simulink library "ammclib_bam_S32K14x"  (R2016a)
settings: Solver=VariableStepAuto  SolverMode=SingleTasking  StartTime=0.0  StopTime=10.0  RelTol=1e-3
undefined symbols (not defined in the file or in its folder): f16A1, f16A2, f16ADCMaxError, f16B0, f16B1, f16B2, f16C1, f16CC1, f16CC1sc, f16CC1sc_D, f16CC1sc_Q, f16CC2, f16CC2sc, f16CC2sc_D, f16CC2sc_Q, f16DerivGain, f16EGain, f16FiltCoef, f16HystOff, f16HystOn, f16IGain, f16IntegGain, f16IntegGainFW, f16IntegGainQ, f16Kd, f16Kq, f16Limit, f16LowerLimit, f16LowerLimit_D, f16LowerLimit_Q, f16LowerLimitFW, f16LowerLimitQ, f16ModIndex, f16OutValOff, f16OutValOn, f16PropGain, f16PropGainFW, f16PropGainQ, f16RampDown, f16RampUp, f16UGain, f16UpperLimit, f16UpperLimit_D, f16UpperLimit_Q, f16UpperLimitFW, f16UpperLimitQ, f16WIGain, f32A1, f32A2, f32ADCMaxError, f32B0, f32B1, f32B2, f32C1, f32CC1, f32CC1sc, f32CC1sc_D, f32CC1sc_Q, f32CC2, f32CC2sc ... (+114)
(part 16 of 22)

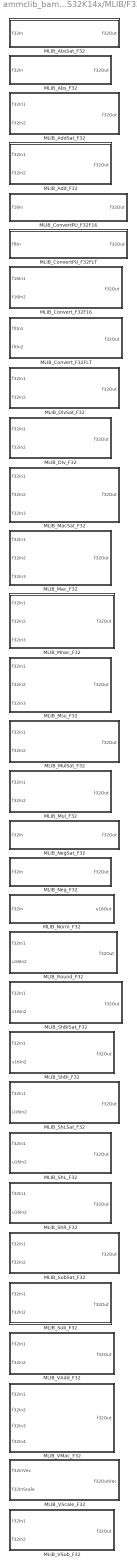
== system ammclib_bam_S32K14x/MLIB/F32 ==
  MLIB_AbsSat_F32 : Subsystem  TreatAsAtomicUnit=on  mask(MLIB_AbsSat_F32){}
      mask help: Saturated absolute value in 32-bit fixed-point fractional implementation. Refer to the AMMCLIB User's Guide for further details.
      mask init: same as ammclib_bam_S32K14x/GDFLIB/F16/GDFLIB_FilterFIR_F16
      settings: RTWSystemCode=Inline
      mask Help: web([fileparts(which('ammclib_bam_S32K14x.slx')) '/../doc/S32K14XMCLUG.pdf'], '-browser')
      mask Display: pos = get_param(gcb, 'Position');width = pos(3) - pos(1); height = pos(4) - pos(2);tX=width/2;tY=height - 8;color('black');text(tX,tY, 'MLIB_AbsSat_F32', 'horizontalAlignment', 'center');
  MLIB_Abs_F32 : Subsystem  TreatAsAtomicUnit=on  mask(MLIB_Abs_F32){}
      mask help: Unsaturated absolute value in 32-bit fixed-point fractional implementation. Refer to the AMMCLIB User's Guide for further details.
      mask init: same as ammclib_bam_S32K14x/GDFLIB/F16/GDFLIB_FilterFIR_F16
      settings: RTWSystemCode=Inline
      mask Help: web([fileparts(which('ammclib_bam_S32K14x.slx')) '/../doc/S32K14XMCLUG.pdf'], '-browser')
      mask Display: pos = get_param(gcb, 'Position');width = pos(3) - pos(1); height = pos(4) - pos(2);tX=width/2;tY=height - 8;color('black');text(tX,tY, 'MLIB_Abs_F32', 'horizontalAlignment', 'center');
  MLIB_AddSat_F32 : Subsystem  TreatAsAtomicUnit=on  mask(MLIB_AddSat_F32){}
      mask help: Saturated addition in 32-bit fixed-point fractional implementation. Refer to the AMMCLIB User's Guide for further details.
      mask init: same as ammclib_bam_S32K14x/GDFLIB/F16/GDFLIB_FilterFIR_F16
      settings: RTWSystemCode=Inline
      mask Help: web([fileparts(which('ammclib_bam_S32K14x.slx')) '/../doc/S32K14XMCLUG.pdf'], '-browser')
      mask Display: pos = get_param(gcb, 'Position');width = pos(3) - pos(1); height = pos(4) - pos(2);tX=width/2;tY=height - 8;color('black');text(tX,tY, 'MLIB_AddSat_F32', 'horizontalAlignment', 'center');
  MLIB_Add_F32 : Subsystem  TreatAsAtomicUnit=on  mask(MLIB_Add_F32){}
      mask help: Unsaturated addition in 32-bit fixed-point fractional implementation.
      mask init: same as ammclib_bam_S32K14x/GDFLIB/F16/GDFLIB_FilterFIR_F16
      settings: RTWSystemCode=Inline
      mask Help: web([fileparts(which('ammclib_bam_S32K14x.slx')) '/../doc/S32K14XMCLUG.pdf'], '-browser')
      mask Display: pos = get_param(gcb, 'Position');width = pos(3) - pos(1); height = pos(4) - pos(2);tX=width/2;tY=height - 8;color('black');text(tX,tY, 'MLIB_Add_F32', 'horizontalAlignment', 'center');
  MLIB_ConvertPU_F32F16 : Subsystem  TreatAsAtomicUnit=on  mask(MLIB_ConvertPU_F32F16){}
      mask help: Conversion of a 16-bit fixed-point fractional value to a 32-bit fixed-point fractional equivalent. Refer to the AMMCLIB User's Guide for further details.
      mask init: same as ammclib_bam_S32K14x/GDFLIB/F16/GDFLIB_FilterFIR_F16
      settings: RTWSystemCode=Inline
      mask Help: web([fileparts(which('ammclib_bam_S32K14x.slx')) '/../doc/S32K14XMCLUG.pdf'], '-browser')
      mask Display: pos = get_param(gcb, 'Position');width = pos(3) - pos(1); height = pos(4) - pos(2);tX=width/2;tY=height - 8;color('black');text(tX,tY, 'MLIB_ConvertPU_F32F16', 'horizontalAlignment', 'center');
  MLIB_ConvertPU_F32FLT : Subsystem  TreatAsAtomicUnit=on  mask(MLIB_ConvertPU_F32FLT){}
      mask help: Conversion of a single precision floating-point value to a 32-bit fixed-point fractional equivalent. Refer to the AMMCLIB User's Guide for further details.
      mask init: same as ammclib_bam_S32K14x/GDFLIB/F16/GDFLIB_FilterFIR_F16
      settings: RTWSystemCode=Inline
      mask Help: web([fileparts(which('ammclib_bam_S32K14x.slx')) '/../doc/S32K14XMCLUG.pdf'], '-browser')
      mask Display: pos = get_param(gcb, 'Position');width = pos(3) - pos(1); height = pos(4) - pos(2);tX=width/2;tY=height - 8;color('black');text(tX,tY, 'MLIB_ConvertPU_F32FLT', 'horizontalAlignment', 'center');
  MLIB_Convert_F32F16 : Subsystem  TreatAsAtomicUnit=on  mask(MLIB_Convert_F32F16){}
      mask help: Scaled conversion of a 16-bit fixed-point fractional value to a 32-bit fixed-point fractional equivalent. Refer to the AMMCLIB User's Guide for further details.
      mask init: same as ammclib_bam_S32K14x/GDFLIB/F16/GDFLIB_FilterFIR_F16
      settings: RTWSystemCode=Inline
      mask Help: web([fileparts(which('ammclib_bam_S32K14x.slx')) '/../doc/S32K14XMCLUG.pdf'], '-browser')
      mask Display: pos = get_param(gcb, 'Position');width = pos(3) - pos(1); height = pos(4) - pos(2);tX=width/2;tY=height - 8;color('black');text(tX,tY, 'MLIB_Convert_F32F16', 'horizontalAlignment', 'center');
  MLIB_Convert_F32FLT : Subsystem  TreatAsAtomicUnit=on  mask(MLIB_Convert_F32FLT){}
      mask help: Scaled conversion of a single precision floating-point value to a 32-bit fixed-point fractional equivalent. Refer to the AMMCLIB User's Guide for further details.
      mask init: same as ammclib_bam_S32K14x/GDFLIB/F16/GDFLIB_FilterFIR_F16
      settings: RTWSystemCode=Inline
      mask Help: web([fileparts(which('ammclib_bam_S32K14x.slx')) '/../doc/S32K14XMCLUG.pdf'], '-browser')
      mask Display: pos = get_param(gcb, 'Position');width = pos(3) - pos(1); height = pos(4) - pos(2);tX=width/2;tY=height - 8;color('black');text(tX,tY, 'MLIB_Convert_F32FLT', 'horizontalAlignment', 'center');
  MLIB_DivSat_F32 : Subsystem  TreatAsAtomicUnit=on  mask(MLIB_DivSat_F32){}
      mask help: Saturated division of two input values in 32-bit fixed-point fractional implementation. Refer to the AMMCLIB User's Guide for further details.
      mask init: same as ammclib_bam_S32K14x/GDFLIB/F16/GDFLIB_FilterFIR_F16
      settings: RTWSystemCode=Inline
      mask Help: web([fileparts(which('ammclib_bam_S32K14x.slx')) '/../doc/S32K14XMCLUG.pdf'], '-browser')
      mask Display: pos = get_param(gcb, 'Position');width = pos(3) - pos(1); height = pos(4) - pos(2);tX=width/2;tY=height - 8;color('black');text(tX,tY, 'MLIB_DivSat_F32', 'horizontalAlignment', 'center');
  MLIB_Div_F32 : Subsystem  TreatAsAtomicUnit=on  mask(MLIB_Div_F32){}
      mask help: Division of two input values without saturation in 32-bit fixed-point fractional implementation. Refer to the AMMCLIB User's Guide for further details.
      mask init: same as ammclib_bam_S32K14x/GDFLIB/F16/GDFLIB_FilterFIR_F16
      settings: RTWSystemCode=Inline
      mask Help: web([fileparts(which('ammclib_bam_S32K14x.slx')) '/../doc/S32K14XMCLUG.pdf'], '-browser')
      mask Display: pos = get_param(gcb, 'Position');width = pos(3) - pos(1); height = pos(4) - pos(2);tX=width/2;tY=height - 8;color('black');text(tX,tY, 'MLIB_Div_F32', 'horizontalAlignment', 'center');
  MLIB_MacSat_F32 : Subsystem  TreatAsAtomicUnit=on  mask(MLIB_MacSat_F32){}
      mask help: Saturated multiply-accumulate of input values in 32-bit fixed-point fractional implementation. Refer to the AMMCLIB User's Guide for further details.
      mask init: same as ammclib_bam_S32K14x/GDFLIB/F16/GDFLIB_FilterFIR_F16
      settings: RTWSystemCode=Inline
      mask Help: web([fileparts(which('ammclib_bam_S32K14x.slx')) '/../doc/S32K14XMCLUG.pdf'], '-browser')
      mask Display: pos = get_param(gcb, 'Position');width = pos(3) - pos(1); height = pos(4) - pos(2);tX=width/2;tY=height - 8;color('black');text(tX,tY, 'MLIB_MacSat_F32', 'horizontalAlignment', 'center');
  MLIB_Mac_F32 : Subsystem  TreatAsAtomicUnit=on  mask(MLIB_Mac_F32){}
      mask help: Unsaturated multiply-accumulate function in 32-bit fixed-point fractional implementation. Refer to the AMMCLIB User's Guide for further details.
      mask init: same as ammclib_bam_S32K14x/GDFLIB/F16/GDFLIB_FilterFIR_F16
      settings: RTWSystemCode=Inline
      mask Help: web([fileparts(which('ammclib_bam_S32K14x.slx')) '/../doc/S32K14XMCLUG.pdf'], '-browser')
      mask Display: pos = get_param(gcb, 'Position');width = pos(3) - pos(1); height = pos(4) - pos(2);tX=width/2;tY=height - 8;color('black');text(tX,tY, 'MLIB_Mac_F32', 'horizontalAlignment', 'center');
  MLIB_Mnac_F32 : Subsystem  TreatAsAtomicUnit=on  mask(MLIB_Mnac_F32){}
      mask help: Unsaturated multiply-negative-accumulate function in 32-bit fixed-point fractional implementation. Refer to the AMMCLIB User's Guide for further details.
      mask init: same as ammclib_bam_S32K14x/GDFLIB/F16/GDFLIB_FilterFIR_F16
      settings: RTWSystemCode=Inline
      mask Help: web([fileparts(which('ammclib_bam_S32K14x.slx')) '/../doc/S32K14XMCLUG.pdf'], '-browser')
      mask Display: pos = get_param(gcb, 'Position');width = pos(3) - pos(1); height = pos(4) - pos(2);tX=width/2;tY=height - 8;color('black');text(tX,tY, 'MLIB_Mnac_F32', 'horizontalAlignment', 'center');
  MLIB_Msu_F32 : Subsystem  TreatAsAtomicUnit=on  mask(MLIB_Msu_F32){}
      mask help: Unsaturated multiply-subtract-from function in 32-bit fixed-point fractional implementation. Refer to the AMMCLIB User's Guide for further details.
      mask init: same as ammclib_bam_S32K14x/GDFLIB/F16/GDFLIB_FilterFIR_F16
      settings: RTWSystemCode=Inline
      mask Help: web([fileparts(which('ammclib_bam_S32K14x.slx')) '/../doc/S32K14XMCLUG.pdf'], '-browser')
      mask Display: pos = get_param(gcb, 'Position');width = pos(3) - pos(1); height = pos(4) - pos(2);tX=width/2;tY=height - 8;color('black');text(tX,tY, 'MLIB_Msu_F32', 'horizontalAlignment', 'center');
  MLIB_MulSat_F32 : Subsystem  TreatAsAtomicUnit=on  mask(MLIB_MulSat_F32){}
      mask help: Saturated multiplication of two input values in 32-bit fixed-point fractional implementation. Refer to the AMMCLIB User's Guide for further details.
      mask init: same as ammclib_bam_S32K14x/GDFLIB/F16/GDFLIB_FilterFIR_F16
      settings: RTWSystemCode=Inline
      mask Help: web([fileparts(which('ammclib_bam_S32K14x.slx')) '/../doc/S32K14XMCLUG.pdf'], '-browser')
      mask Display: pos = get_param(gcb, 'Position');width = pos(3) - pos(1); height = pos(4) - pos(2);tX=width/2;tY=height - 8;color('black');text(tX,tY, 'MLIB_MulSat_F32', 'horizontalAlignment', 'center');
  MLIB_Mul_F32 : Subsystem  TreatAsAtomicUnit=on  mask(MLIB_Mul_F32){}
      mask help: Unsaturated multiplication of two input values in 32-bit fixed-point fractional implementation. Refer to the AMMCLIB User's Guide for further details.
      mask init: same as ammclib_bam_S32K14x/GDFLIB/F16/GDFLIB_FilterFIR_F16
      settings: RTWSystemCode=Inline
      mask Help: web([fileparts(which('ammclib_bam_S32K14x.slx')) '/../doc/S32K14XMCLUG.pdf'], '-browser')
      mask Display: pos = get_param(gcb, 'Position');width = pos(3) - pos(1); height = pos(4) - pos(2);tX=width/2;tY=height - 8;color('black');text(tX,tY, 'MLIB_Mul_F32', 'horizontalAlignment', 'center');
  MLIB_NegSat_F32 : Subsystem  TreatAsAtomicUnit=on  mask(MLIB_NegSat_F32){}
      mask help: Saturated negation in 32-bit fixed-point fractional implementation. Refer to the AMMCLIB User's Guide for further details.
      mask init: same as ammclib_bam_S32K14x/GDFLIB/F16/GDFLIB_FilterFIR_F16
      settings: RTWSystemCode=Inline
      mask Help: web([fileparts(which('ammclib_bam_S32K14x.slx')) '/../doc/S32K14XMCLUG.pdf'], '-browser')
      mask Display: pos = get_param(gcb, 'Position');width = pos(3) - pos(1); height = pos(4) - pos(2);tX=width/2;tY=height - 8;color('black');text(tX,tY, 'MLIB_NegSat_F32', 'horizontalAlignment', 'center');
  MLIB_Neg_F32 : Subsystem  TreatAsAtomicUnit=on  mask(MLIB_Neg_F32){}
      mask help: Unsaturated negation in 32-bit fixed-point fractional implementation. Refer to the AMMCLIB User's Guide for further details.
      mask init: same as ammclib_bam_S32K14x/GDFLIB/F16/GDFLIB_FilterFIR_F16
      settings: RTWSystemCode=Inline
      mask Help: web([fileparts(which('ammclib_bam_S32K14x.slx')) '/../doc/S32K14XMCLUG.pdf'], '-browser')
      mask Display: pos = get_param(gcb, 'Position');width = pos(3) - pos(1); height = pos(4) - pos(2);tX=width/2;tY=height - 8;color('black');text(tX,tY, 'MLIB_Neg_F32', 'horizontalAlignment', 'center');
  MLIB_Norm_F32 : Subsystem  TreatAsAtomicUnit=on  mask(MLIB_Norm_F32){}
      mask help: Normalization function in 32-bit fixed-point fractional implementation. The function counts the number of left shift needed for normalization of the input fractional value. Refer to the AMMCLIB User's Guide for further details.
      mask init: same as ammclib_bam_S32K14x/GDFLIB/F16/GDFLIB_FilterFIR_F16
      settings: RTWSystemCode=Inline
      mask Help: web([fileparts(which('ammclib_bam_S32K14x.slx')) '/../doc/S32K14XMCLUG.pdf'], '-browser')
      mask Display: pos = get_param(gcb, 'Position');width = pos(3) - pos(1); height = pos(4) - pos(2);tX=width/2;tY=height - 8;color('black');text(tX,tY, 'MLIB_Norm_F32', 'horizontalAlignment', 'center');
  MLIB_Round_F32 : Subsystem  TreatAsAtomicUnit=on  mask(MLIB_Round_F32){}
      mask help: Rounding function in 32-bit fixed-point fractional implementation. The function rounds the first input value to the number of digits defined by second input value and saturates the result. Refer to the AMMCLIB User's Guide for further details.
      mask init: same as ammclib_bam_S32K14x/GDFLIB/F16/GDFLIB_FilterFIR_F16
      settings: RTWSystemCode=Inline
      mask Help: web([fileparts(which('ammclib_bam_S32K14x.slx')) '/../doc/S32K14XMCLUG.pdf'], '-browser')
      mask Display: pos = get_param(gcb, 'Position');width = pos(3) - pos(1); height = pos(4) - pos(2);tX=width/2;tY=height - 8;color('black');text(tX,tY, 'MLIB_Round_F32', 'horizontalAlignment', 'center');
  MLIB_ShBiSat_F32 : Subsystem  TreatAsAtomicUnit=on  mask(MLIB_ShBiSat_F32){}
      mask help: Saturated bidirectional shift in 32-bit fixed-point fractional implementation. The function shifts the first input value to the left (if the second input is negative) or right (if the second input is positive) by the amount defined by second input value, saturating the result. Refer to the AMMCLIB User's Guide for further details.
      mask init: same as ammclib_bam_S32K14x/GDFLIB/F16/GDFLIB_FilterFIR_F16
      settings: RTWSystemCode=Inline
      mask Help: web([fileparts(which('ammclib_bam_S32K14x.slx')) '/../doc/S32K14XMCLUG.pdf'], '-browser')
      mask Display: pos = get_param(gcb, 'Position');width = pos(3) - pos(1); height = pos(4) - pos(2);tX=width/2;tY=height - 8;color('black');text(tX,tY, 'MLIB_ShBiSat_F32', 'horizontalAlignment', 'center');
  MLIB_ShBi_F32 : Subsystem  TreatAsAtomicUnit=on  mask(MLIB_ShBi_F32){}
      mask help: Unsaturated bidirectional shift in 32-bit fixed-point fractional implementation. The function shifts the first input value to the left (if the second input is negative) or right (if the second input is positive) by the amount defined by second input value. Refer to the AMMCLIB User's Guide for further details.
      mask init: same as ammclib_bam_S32K14x/GDFLIB/F16/GDFLIB_FilterFIR_F16
      settings: RTWSystemCode=Inline
      mask Help: web([fileparts(which('ammclib_bam_S32K14x.slx')) '/../doc/S32K14XMCLUG.pdf'], '-browser')
      mask Display: pos = get_param(gcb, 'Position');width = pos(3) - pos(1); height = pos(4) - pos(2);tX=width/2;tY=height - 8;color('black');text(tX,tY, 'MLIB_ShBi_F32', 'horizontalAlignment', 'center');
  MLIB_ShLSat_F32 : Subsystem  TreatAsAtomicUnit=on  mask(MLIB_ShLSat_F32){}
      mask help: Saturated shift left in 32-bit fixed-point fractional implementation. The function shifts the first input value to the left by the amount defined by the second input value, saturating the result. Refer to the AMMCLIB User's Guide for further details.
      mask init: same as ammclib_bam_S32K14x/GDFLIB/F16/GDFLIB_FilterFIR_F16
      settings: RTWSystemCode=Inline
      mask Help: web([fileparts(which('ammclib_bam_S32K14x.slx')) '/../doc/S32K14XMCLUG.pdf'], '-browser')
      mask Display: pos = get_param(gcb, 'Position');width = pos(3) - pos(1); height = pos(4) - pos(2);tX=width/2;tY=height - 8;color('black');text(tX,tY, 'MLIB_ShLSat_F32', 'horizontalAlignment', 'center');
  MLIB_ShL_F32 : Subsystem  TreatAsAtomicUnit=on  mask(MLIB_ShL_F32){}
      mask help: Unsaturated shift left in 32-bit fixed-point fractional implementation. The function shifts the first input value to the left by the amount defined by the second input value. Refer to the AMMCLIB User's Guide for further details.
      mask init: same as ammclib_bam_S32K14x/GDFLIB/F16/GDFLIB_FilterFIR_F16
      settings: RTWSystemCode=Inline
      mask Help: web([fileparts(which('ammclib_bam_S32K14x.slx')) '/../doc/S32K14XMCLUG.pdf'], '-browser')
      mask Display: pos = get_param(gcb, 'Position');width = pos(3) - pos(1); height = pos(4) - pos(2);tX=width/2;tY=height - 8;color('black');text(tX,tY, 'MLIB_ShL_F32', 'horizontalAlignment', 'center');
  MLIB_ShR_F32 : Subsystem  TreatAsAtomicUnit=on  mask(MLIB_ShR_F32){}
      mask help: Unsaturated shift right in 32-bit fixed-point fractional implementation. The function shifts the first input value to the right by the amount defined by the second input value. Refer to the AMMCLIB User's Guide for further details.
      mask init: same as ammclib_bam_S32K14x/GDFLIB/F16/GDFLIB_FilterFIR_F16
      settings: RTWSystemCode=Inline
      mask Help: web([fileparts(which('ammclib_bam_S32K14x.slx')) '/../doc/S32K14XMCLUG.pdf'], '-browser')
      mask Display: pos = get_param(gcb, 'Position');width = pos(3) - pos(1); height = pos(4) - pos(2);tX=width/2;tY=height - 8;color('black');text(tX,tY, 'MLIB_ShR_F32', 'horizontalAlignment', 'center');
  MLIB_SubSat_F32 : Subsystem  TreatAsAtomicUnit=on  mask(MLIB_SubSat_F32){}
      mask help: Saturated subtraction in 32-bit fixed-point fractional implementation. Refer to the AMMCLIB User's Guide for further details.
      mask init: same as ammclib_bam_S32K14x/GDFLIB/F16/GDFLIB_FilterFIR_F16
      settings: RTWSystemCode=Inline
      mask Help: web([fileparts(which('ammclib_bam_S32K14x.slx')) '/../doc/S32K14XMCLUG.pdf'], '-browser')
      mask Display: pos = get_param(gcb, 'Position');width = pos(3) - pos(1); height = pos(4) - pos(2);tX=width/2;tY=height - 8;color('black');text(tX,tY, 'MLIB_SubSat_F32', 'horizontalAlignment', 'center');
  MLIB_Sub_F32 : Subsystem  TreatAsAtomicUnit=on  mask(MLIB_Sub_F32){}
      mask help: Unsaturated subtraction in 32-bit fixed-point fractional implementation. Refer to the AMMCLIB User's Guide for further details.
      mask init: same as ammclib_bam_S32K14x/GDFLIB/F16/GDFLIB_FilterFIR_F16
      settings: RTWSystemCode=Inline
      mask Help: web([fileparts(which('ammclib_bam_S32K14x.slx')) '/../doc/S32K14XMCLUG.pdf'], '-browser')
      mask Display: pos = get_param(gcb, 'Position');width = pos(3) - pos(1); height = pos(4) - pos(2);tX=width/2;tY=height - 8;color('black');text(tX,tY, 'MLIB_Sub_F32', 'horizontalAlignment', 'center');
  MLIB_VAdd_F32 : Subsystem  TreatAsAtomicUnit=on  mask(MLIB_VAdd_F32){}
      mask help: Vector addition in 32-bit fixed-point fractional implementation.
      mask init: same as ammclib_bam_S32K14x/GDFLIB/F16/GDFLIB_FilterFIR_F16
      settings: RTWSystemCode=Inline
      mask Help: web([fileparts(which('ammclib_bam_S32K14x.slx')) '/../doc/S32K14XMCLUG.pdf'], '-browser')
      mask Display: pos = get_param(gcb, 'Position');width = pos(3) - pos(1); height = pos(4) - pos(2);tX=width/2;tY=height - 8;color('black');text(tX,tY, 'MLIB_VAdd_F32', 'horizontalAlignment', 'center');
  MLIB_VMac_F32 : Subsystem  TreatAsAtomicUnit=on  mask(MLIB_VMac_F32){}
      mask help: Dot product of 2-element vectors with saturated multiplication and modulo accumulation in 32-bit fixed-point fractional implementation. Refer to the AMMCLIB User's Guide for further details.
      mask init: same as ammclib_bam_S32K14x/GDFLIB/F16/GDFLIB_FilterFIR_F16
      settings: RTWSystemCode=Inline
      mask Help: web([fileparts(which('ammclib_bam_S32K14x.slx')) '/../doc/S32K14XMCLUG.pdf'], '-browser')
      mask Display: pos = get_param(gcb, 'Position');width = pos(3) - pos(1); height = pos(4) - pos(2);tX=width/2;tY=height - 8;color('black');text(tX,tY, 'MLIB_VMac_F32', 'horizontalAlignment', 'center');
  MLIB_VScale_F32 : Subsystem  TreatAsAtomicUnit=on  mask(MLIB_VScale_F32){}
      mask help: Multiplication of a vector and scalar in 32-bit fixed-point fractional implementation.
      mask init: same as ammclib_bam_S32K14x/GDFLIB/F16/GDFLIB_FilterFIR_F16
      settings: RTWSystemCode=Inline
      mask Help: web([fileparts(which('ammclib_bam_S32K14x.slx')) '/../doc/S32K14XMCLUG.pdf'], '-browser')
      mask Display: pos = get_param(gcb, 'Position');width = pos(3) - pos(1); height = pos(4) - pos(2);tX=width/2;tY=height - 8;color('black');text(tX,tY, 'MLIB_VScale_F32', 'horizontalAlignment', 'center');
  MLIB_VSub_F32 : Subsystem  TreatAsAtomicUnit=on  mask(MLIB_VSub_F32){}
      mask help: Vector substraction in 32-bit fixed-point fractional implementation.
      mask init: same as ammclib_bam_S32K14x/GDFLIB/F16/GDFLIB_FilterFIR_F16
      settings: RTWSystemCode=Inline
      mask Help: web([fileparts(which('ammclib_bam_S32K14x.slx')) '/../doc/S32K14XMCLUG.pdf'], '-browser')
      mask Display: pos = get_param(gcb, 'Position');width = pos(3) - pos(1); height = pos(4) - pos(2);tX=width/2;tY=height - 8;color('black');text(tX,tY, 'MLIB_VSub_F32', 'horizontalAlignment', 'center');

== system ammclib_bam_S32K14x/MLIB/F32F16F16 ==
  MLIB_MacSat_F32F16F16 : Subsystem  TreatAsAtomicUnit=on  mask(MLIB_MacSat_F32F16F16){}
      mask help: Saturated multiply-accumulate of input values in 16/32-bit fixed-point fractional implementation. Refer to the AMMCLIB User's Guide for further details.
      mask init: same as ammclib_bam_S32K14x/GDFLIB/F16/GDFLIB_FilterFIR_F16
      settings: RTWSystemCode=Inline
      mask Help: web([fileparts(which('ammclib_bam_S32K14x.slx')) '/../doc/S32K14XMCLUG.pdf'], '-browser')
      mask Display: pos = get_param(gcb, 'Position');width = pos(3) - pos(1); height = pos(4) - pos(2);tX=width/2;tY=height - 8;color('black');text(tX,tY, 'MLIB_MacSat_F32F16F16', 'horizontalAlignment', 'center');
  MLIB_Mac_F32F16F16 : Subsystem  TreatAsAtomicUnit=on  mask(MLIB_Mac_F32F16F16){}
      mask help: Unsaturated multiply-accumulate function in 16/32-bit fixed-point fractional implementation. Refer to the AMMCLIB User's Guide for further details.
      mask init: same as ammclib_bam_S32K14x/GDFLIB/F16/GDFLIB_FilterFIR_F16
      settings: RTWSystemCode=Inline
      mask Help: web([fileparts(which('ammclib_bam_S32K14x.slx')) '/../doc/S32K14XMCLUG.pdf'], '-browser')
      mask Display: pos = get_param(gcb, 'Position');width = pos(3) - pos(1); height = pos(4) - pos(2);tX=width/2;tY=height - 8;color('black');text(tX,tY, 'MLIB_Mac_F32F16F16', 'horizontalAlignment', 'center');
  MLIB_Mnac_F32F16F16 : Subsystem  TreatAsAtomicUnit=on  mask(MLIB_Mnac_F32F16F16){}
      mask help: Unsaturated multiply-negative-accumulate function in 16/32-bit fixed-point fractional implementation. Refer to the AMMCLIB User's Guide for further details.
      mask init: same as ammclib_bam_S32K14x/GDFLIB/F16/GDFLIB_FilterFIR_F16
      settings: RTWSystemCode=Inline
      mask Help: web([fileparts(which('ammclib_bam_S32K14x.slx')) '/../doc/S32K14XMCLUG.pdf'], '-browser')
      mask Display: pos = get_param(gcb, 'Position');width = pos(3) - pos(1); height = pos(4) - pos(2);tX=width/2;tY=height - 8;color('black');text(tX,tY, 'MLIB_Mnac_F32F16F16', 'horizontalAlignment', 'center');
  MLIB_Msu_F32F16F16 : Subsystem  TreatAsAtomicUnit=on  mask(MLIB_Msu_F32F16F16){}
      mask help: Unsaturated multiply-subtract-from function in 16/32-bit fixed-point fractional implementation. Refer to the AMMCLIB User's Guide for further details.
      mask init: same as ammclib_bam_S32K14x/GDFLIB/F16/GDFLIB_FilterFIR_F16
      settings: RTWSystemCode=Inline
      mask Help: web([fileparts(which('ammclib_bam_S32K14x.slx')) '/../doc/S32K14XMCLUG.pdf'], '-browser')
      mask Display: pos = get_param(gcb, 'Position');width = pos(3) - pos(1); height = pos(4) - pos(2);tX=width/2;tY=height - 8;color('black');text(tX,tY, 'MLIB_Msu_F32F16F16', 'horizontalAlignment', 'center');
  MLIB_MulSat_F32F16F16 : Subsystem  TreatAsAtomicUnit=on  mask(MLIB_MulSat_F32F16F16){}
      mask help: Saturated multiplication of two input values in 16/32-bit fixed-point fractional implementation. Refer to the AMMCLIB User's Guide for further details.
      mask init: same as ammclib_bam_S32K14x/GDFLIB/F16/GDFLIB_FilterFIR_F16
      settings: RTWSystemCode=Inline
      mask Help: web([fileparts(which('ammclib_bam_S32K14x.slx')) '/../doc/S32K14XMCLUG.pdf'], '-browser')
      mask Display: pos = get_param(gcb, 'Position');width = pos(3) - pos(1); height = pos(4) - pos(2);tX=width/2;tY=height - 8;color('black');text(tX,tY, 'MLIB_MulSat_F32F16F16', 'horizontalAlignment', 'center');
  MLIB_Mul_F32F16F16 : Subsystem  TreatAsAtomicUnit=on  mask(MLIB_Mul_F32F16F16){}
      mask help: Unsaturated multiplication of two input values in 16/32-bit fixed-point fractional implementation. Refer to the AMMCLIB User's Guide for further details.
      mask init: same as ammclib_bam_S32K14x/GDFLIB/F16/GDFLIB_FilterFIR_F16
      settings: RTWSystemCode=Inline
      mask Help: web([fileparts(which('ammclib_bam_S32K14x.slx')) '/../doc/S32K14XMCLUG.pdf'], '-browser')
      mask Display: pos = get_param(gcb, 'Position');width = pos(3) - pos(1); height = pos(4) - pos(2);tX=width/2;tY=height - 8;color('black');text(tX,tY, 'MLIB_Mul_F32F16F16', 'horizontalAlignment', 'center');
  MLIB_VMac_F32F16F16 : Subsystem  TreatAsAtomicUnit=on  mask(MLIB_VMac_F32F16F16){}
      mask help: Dot product of 2-element vectors with saturated multiplication and modulo accumulation in 16/32-bit fixed-point fractional implementation. Refer to the AMMCLIB User's Guide for further details.
      mask init: same as ammclib_bam_S32K14x/GDFLIB/F16/GDFLIB_FilterFIR_F16
      settings: RTWSystemCode=Inline
      mask Help: web([fileparts(which('ammclib_bam_S32K14x.slx')) '/../doc/S32K14XMCLUG.pdf'], '-browser')
      mask Display: pos = get_param(gcb, 'Position');width = pos(3) - pos(1); height = pos(4) - pos(2);tX=width/2;tY=height - 8;color('black');text(tX,tY, 'MLIB_VMac_F32F16F16', 'horizontalAlignment', 'center');

== system ammclib_bam_S32K14x/MLIB/FLT ==
  MLIB_Abs_FLT : Subsystem  TreatAsAtomicUnit=on  mask(MLIB_Abs_FLT){}
      mask help: Absolute value in single precision floating-point implementation. Refer to the AMMCLIB User's Guide for further details.
      mask init: same as ammclib_bam_S32K14x/GDFLIB/F16/GDFLIB_FilterFIR_F16
      settings: RTWSystemCode=Inline
      mask Help: web([fileparts(which('ammclib_bam_S32K14x.slx')) '/../doc/S32K14XMCLUG.pdf'], '-browser')
      mask Display: pos = get_param(gcb, 'Position');width = pos(3) - pos(1); height = pos(4) - pos(2);tX=width/2;tY=height - 8;color('black');text(tX,tY, 'MLIB_Abs_FLT', 'horizontalAlignment', 'center');
  MLIB_Add_FLT : Subsystem  TreatAsAtomicUnit=on  mask(MLIB_Add_FLT){}
      mask help: Addition in single precision floating-point implementation.
      mask init: same as ammclib_bam_S32K14x/GDFLIB/F16/GDFLIB_FilterFIR_F16
      settings: RTWSystemCode=Inline
      mask Help: web([fileparts(which('ammclib_bam_S32K14x.slx')) '/../doc/S32K14XMCLUG.pdf'], '-browser')
      mask Display: pos = get_param(gcb, 'Position');width = pos(3) - pos(1); height = pos(4) - pos(2);tX=width/2;tY=height - 8;color('black');text(tX,tY, 'MLIB_Add_FLT', 'horizontalAlignment', 'center');
  MLIB_ConvertPU_FLTF16 : Subsystem  TreatAsAtomicUnit=on  mask(MLIB_ConvertPU_FLTF16){}
      mask help: Conversion of a 16-bit fixed-point fractional value to a single precision floating-point equivalent. Refer to the AMMCLIB User's Guide for further details.
      mask init: same as ammclib_bam_S32K14x/GDFLIB/F16/GDFLIB_FilterFIR_F16
      settings: RTWSystemCode=Inline
      mask Help: web([fileparts(which('ammclib_bam_S32K14x.slx')) '/../doc/S32K14XMCLUG.pdf'], '-browser')
      mask Display: pos = get_param(gcb, 'Position');width = pos(3) - pos(1); height = pos(4) - pos(2);tX=width/2;tY=height - 8;color('black');text(tX,tY, 'MLIB_ConvertPU_FLTF16', 'horizontalAlignment', 'center');
  MLIB_ConvertPU_FLTF32 : Subsystem  TreatAsAtomicUnit=on  mask(MLIB_ConvertPU_FLTF32){}
      mask help: Conversion of a 32-bit fixed-point fractional value to a single precision floating-point equivalent. Refer to the AMMCLIB User's Guide for further details.
      mask init: same as ammclib_bam_S32K14x/GDFLIB/F16/GDFLIB_FilterFIR_F16
      settings: RTWSystemCode=Inline
      mask Help: web([fileparts(which('ammclib_bam_S32K14x.slx')) '/../doc/S32K14XMCLUG.pdf'], '-browser')
      mask Display: pos = get_param(gcb, 'Position');width = pos(3) - pos(1); height = pos(4) - pos(2);tX=width/2;tY=height - 8;color('black');text(tX,tY, 'MLIB_ConvertPU_FLTF32', 'horizontalAlignment', 'center');
  MLIB_Convert_FLTF16 : Subsystem  TreatAsAtomicUnit=on  mask(MLIB_Convert_FLTF16){}
      mask help: Scaled conversion of a 16-bit fixed-point fractional value to a single precision floating-point equivalent. Refer to the AMMCLIB User's Guide for further details.
      mask init: same as ammclib_bam_S32K14x/GDFLIB/F16/GDFLIB_FilterFIR_F16
      settings: RTWSystemCode=Inline
      mask Help: web([fileparts(which('ammclib_bam_S32K14x.slx')) '/../doc/S32K14XMCLUG.pdf'], '-browser')
      mask Display: pos = get_param(gcb, 'Position');width = pos(3) - pos(1); height = pos(4) - pos(2);tX=width/2;tY=height - 8;color('black');text(tX,tY, 'MLIB_Convert_FLTF16', 'horizontalAlignment', 'center');
  MLIB_Convert_FLTF32 : Subsystem  TreatAsAtomicUnit=on  mask(MLIB_Convert_FLTF32){}
      mask help: Scaled conversion of a 32-bit fixed-point fractional value to a single precision floating-point equivalent. Refer to the AMMCLIB User's Guide for further details.
      mask init: same as ammclib_bam_S32K14x/GDFLIB/F16/GDFLIB_FilterFIR_F16
      settings: RTWSystemCode=Inline
      mask Help: web([fileparts(which('ammclib_bam_S32K14x.slx')) '/../doc/S32K14XMCLUG.pdf'], '-browser')
      mask Display: pos = get_param(gcb, 'Position');width = pos(3) - pos(1); height = pos(4) - pos(2);tX=width/2;tY=height - 8;color('black');text(tX,tY, 'MLIB_Convert_FLTF32', 'horizontalAlignment', 'center');
  MLIB_Div_FLT : Subsystem  TreatAsAtomicUnit=on  mask(MLIB_Div_FLT){}
      mask help: Division of two input values in single precision floating-point implementation. Refer to the AMMCLIB User's Guide for further details.
      mask init: same as ammclib_bam_S32K14x/GDFLIB/F16/GDFLIB_FilterFIR_F16
      settings: RTWSystemCode=Inline
      mask Help: web([fileparts(which('ammclib_bam_S32K14x.slx')) '/../doc/S32K14XMCLUG.pdf'], '-browser')
      mask Display: pos = get_param(gcb, 'Position');width = pos(3) - pos(1); height = pos(4) - pos(2);tX=width/2;tY=height - 8;color('black');text(tX,tY, 'MLIB_Div_FLT', 'horizontalAlignment', 'center');
  MLIB_Mac_FLT : Subsystem  TreatAsAtomicUnit=on  mask(MLIB_Mac_FLT){}
      mask help: Multiply accumulate function in single precision floating-point implementation. Refer to the AMMCLIB User's Guide for further details.
      mask init: same as ammclib_bam_S32K14x/GDFLIB/F16/GDFLIB_FilterFIR_F16
      settings: RTWSystemCode=Inline
      mask Help: web([fileparts(which('ammclib_bam_S32K14x.slx')) '/../doc/S32K14XMCLUG.pdf'], '-browser')
      mask Display: pos = get_param(gcb, 'Position');width = pos(3) - pos(1); height = pos(4) - pos(2);tX=width/2;tY=height - 8;color('black');text(tX,tY, 'MLIB_Mac_FLT', 'horizontalAlignment', 'center');
  MLIB_Mnac_FLT : Subsystem  TreatAsAtomicUnit=on  mask(MLIB_Mnac_FLT){}
      mask help: Multiply-negative-accumulate function in 32-bit fixed-point fractional implementation. Refer to the AMMCLIB User's Guide for further details.
      mask init: same as ammclib_bam_S32K14x/GDFLIB/F16/GDFLIB_FilterFIR_F16
      settings: RTWSystemCode=Inline
      mask Help: web([fileparts(which('ammclib_bam_S32K14x.slx')) '/../doc/S32K14XMCLUG.pdf'], '-browser')
      mask Display: pos = get_param(gcb, 'Position');width = pos(3) - pos(1); height = pos(4) - pos(2);tX=width/2;tY=height - 8;color('black');text(tX,tY, 'MLIB_Mnac_FLT', 'horizontalAlignment', 'center');
  MLIB_Msu_FLT : Subsystem  TreatAsAtomicUnit=on  mask(MLIB_Msu_FLT){}
      mask help: Multiply-subtract-from function in single precision floating-point implementation. Refer to the AMMCLIB User's Guide for further details.
      mask init: same as ammclib_bam_S32K14x/GDFLIB/F16/GDFLIB_FilterFIR_F16
      settings: RTWSystemCode=Inline
      mask Help: web([fileparts(which('ammclib_bam_S32K14x.slx')) '/../doc/S32K14XMCLUG.pdf'], '-browser')
      mask Display: pos = get_param(gcb, 'Position');width = pos(3) - pos(1); height = pos(4) - pos(2);tX=width/2;tY=height - 8;color('black');text(tX,tY, 'MLIB_Msu_FLT', 'horizontalAlignment', 'center');
  MLIB_Mul_FLT : Subsystem  TreatAsAtomicUnit=on  mask(MLIB_Mul_FLT){}
      mask help: Multiplication of two input values in single precision floating-point implementation. Refer to the AMMCLIB User's Guide for further details.
      mask init: same as ammclib_bam_S32K14x/GDFLIB/F16/GDFLIB_FilterFIR_F16
      settings: RTWSystemCode=Inline
      mask Help: web([fileparts(which('ammclib_bam_S32K14x.slx')) '/../doc/S32K14XMCLUG.pdf'], '-browser')
      mask Display: pos = get_param(gcb, 'Position');width = pos(3) - pos(1); height = pos(4) - pos(2);tX=width/2;tY=height - 8;color('black');text(tX,tY, 'MLIB_Mul_FLT', 'horizontalAlignment', 'center');
  MLIB_Neg_FLT : Subsystem  TreatAsAtomicUnit=on  mask(MLIB_Neg_FLT){}
      mask help: Negation in single precision floating-point implementation. Refer to the AMMCLIB User's Guide for further details.
      mask init: same as ammclib_bam_S32K14x/GDFLIB/F16/GDFLIB_FilterFIR_F16
      settings: RTWSystemCode=Inline
      mask Help: web([fileparts(which('ammclib_bam_S32K14x.slx')) '/../doc/S32K14XMCLUG.pdf'], '-browser')
      mask Display: pos = get_param(gcb, 'Position');width = pos(3) - pos(1); height = pos(4) - pos(2);tX=width/2;tY=height - 8;color('black');text(tX,tY, 'MLIB_Neg_FLT', 'horizontalAlignment', 'center');
  MLIB_Sub_FLT : Subsystem  TreatAsAtomicUnit=on  mask(MLIB_Sub_FLT){}
      mask help: Subtraction in single precision floating-point implementation. Refer to the AMMCLIB User's Guide for further details.
      mask init: same as ammclib_bam_S32K14x/GDFLIB/F16/GDFLIB_FilterFIR_F16
      settings: RTWSystemCode=Inline
      mask Help: web([fileparts(which('ammclib_bam_S32K14x.slx')) '/../doc/S32K14XMCLUG.pdf'], '-browser')
      mask Display: pos = get_param(gcb, 'Position');width = pos(3) - pos(1); height = pos(4) - pos(2);tX=width/2;tY=height - 8;color('black');text(tX,tY, 'MLIB_Sub_FLT', 'horizontalAlignment', 'center');
  MLIB_VAdd_FLT : Subsystem  TreatAsAtomicUnit=on  mask(MLIB_VAdd_FLT){}
      mask help: Vector addition in single precision floating-point implementation.
      mask init: same as ammclib_bam_S32K14x/GDFLIB/F16/GDFLIB_FilterFIR_F16
      settings: RTWSystemCode=Inline
      mask Help: web([fileparts(which('ammclib_bam_S32K14x.slx')) '/../doc/S32K14XMCLUG.pdf'], '-browser')
      mask Display: pos = get_param(gcb, 'Position');width = pos(3) - pos(1); height = pos(4) - pos(2);tX=width/2;tY=height - 8;color('black');text(tX,tY, 'MLIB_VAdd_FLT', 'horizontalAlignment', 'center');
  MLIB_VMac_FLT : Subsystem  TreatAsAtomicUnit=on  mask(MLIB_VMac_FLT){}
      mask help: Dot product of 2-element vectors in single precision floating-point implementation. Refer to the AMMCLIB User's Guide for further details.
      mask init: same as ammclib_bam_S32K14x/GDFLIB/F16/GDFLIB_FilterFIR_F16
      settings: RTWSystemCode=Inline
      mask Help: web([fileparts(which('ammclib_bam_S32K14x.slx')) '/../doc/S32K14XMCLUG.pdf'], '-browser')
      mask Display: pos = get_param(gcb, 'Position');width = pos(3) - pos(1); height = pos(4) - pos(2);tX=width/2;tY=height - 8;color('black');text(tX,tY, 'MLIB_VMac_FLT', 'horizontalAlignment', 'center');
  MLIB_VScale_FLT : Subsystem  TreatAsAtomicUnit=on  mask(MLIB_VScale_FLT){}
      mask help: Multiplication of a vector and scalar in single precision floating-point implementation.
      mask init: same as ammclib_bam_S32K14x/GDFLIB/F16/GDFLIB_FilterFIR_F16
      settings: RTWSystemCode=Inline
      mask Help: web([fileparts(which('ammclib_bam_S32K14x.slx')) '/../doc/S32K14XMCLUG.pdf'], '-browser')
      mask Display: pos = get_param(gcb, 'Position');width = pos(3) - pos(1); height = pos(4) - pos(2);tX=width/2;tY=height - 8;color('black');text(tX,tY, 'MLIB_VScale_FLT', 'horizontalAlignment', 'center');
  MLIB_VSub_FLT : Subsystem  TreatAsAtomicUnit=on  mask(MLIB_VSub_FLT){}
      mask help: Vector substraction in single precision floating-point implementation.
      mask init: same as ammclib_bam_S32K14x/GDFLIB/F16/GDFLIB_FilterFIR_F16
      settings: RTWSystemCode=Inline
      mask Help: web([fileparts(which('ammclib_bam_S32K14x.slx')) '/../doc/S32K14XMCLUG.pdf'], '-browser')
      mask Display: pos = get_param(gcb, 'Position');width = pos(3) - pos(1); height = pos(4) - pos(2);tX=width/2;tY=height - 8;color('black');text(tX,tY, 'MLIB_VSub_FLT', 'horizontalAlignment', 'center');

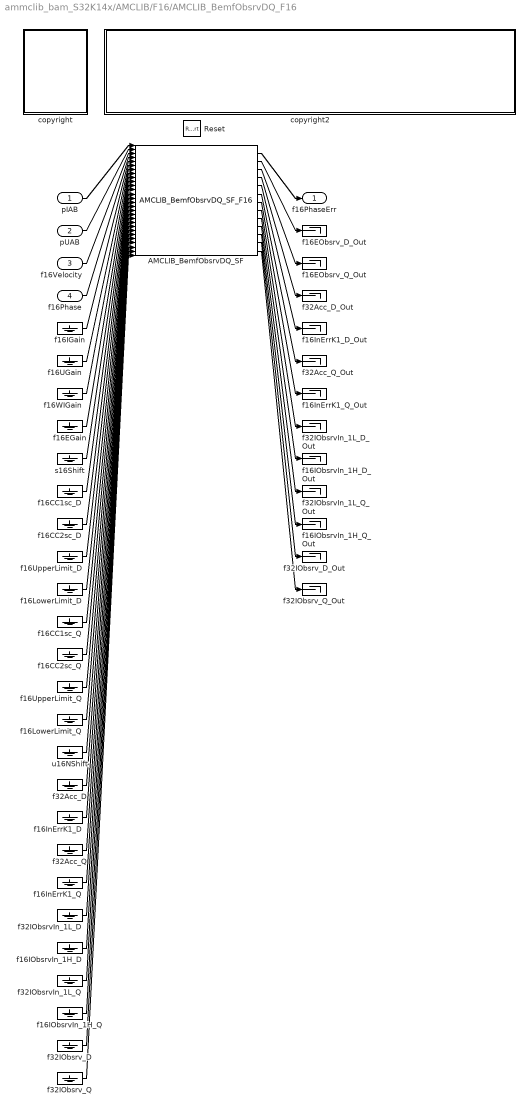
== system ammclib_bam_S32K14x/AMCLIB/F16/AMCLIB_BemfObsrvDQ_F16 ==
  pIAB : Inport  OutDataTypeStr=Bus: SWLIBS_2Syst_F16  BusOutputAsStruct=on
  pUAB : Inport  Port=2  OutDataTypeStr=Bus: SWLIBS_2Syst_F16  BusOutputAsStruct=on
  f16Velocity : Inport  Port=3  OutDataTypeStr=int16
  f16Phase : Inport  Port=4  OutDataTypeStr=int16
  Reset : ResetPort  DisableCoverage=on
  AMCLIB_BemfObsrvDQ_SF : S-Function  FunctionName=AMCLIB_BemfObsrvDQ_SF_F16  Parameters=showStates,resetStatesEnable,f16IGain,f16UGain,f16WIGain,f16EGain,s16Shift,f16CC1sc_D,f16CC2sc_D,f16UpperLimit_D,f16LowerLimit_D,f16CC1sc_Q,f16CC2sc_Q,f16UpperLimit_Q,f16LowerLimit_Q,u16NShift  SFunctionDeploymentMode=off  EnableBusSupport=off
  copyright : Subsystem
      mask Display: text(10,90,'FILE:');text(10,75,'DESRIPTION:');text(10,60,'COPYRIGHT:');text(10,45,'VERSION:');text(10,30,'DATE:')
  copyright2 : Subsystem
      mask Display: text(10,90,'AMCLIB_BemfObsrvDQ_BAM_F16.mdl');text(10,75,'PMSM back-EMF observer DQ.');text(10,60,'NXP 2020');text(10,45,'1.0');text(10,30,'28-Mar-2020');
  f16CC1sc_D : Ground
  f16CC1sc_Q : Ground
  f16CC2sc_D : Ground
  f16CC2sc_Q : Ground
  f16EGain : Ground
  f16EObsrv_D_Out : Terminator
  f16EObsrv_Q_Out : Terminator
  f16IGain : Ground
  f16IObsrvIn_1H_D : Ground
  f16IObsrvIn_1H_D_Out : Terminator
  f16IObsrvIn_1H_Q : Ground
  f16IObsrvIn_1H_Q_Out : Terminator
  f16InErrK1_D : Ground
  f16InErrK1_D_Out : Terminator
  f16InErrK1_Q : Ground
  f16InErrK1_Q_Out : Terminator
  f16LowerLimit_D : Ground
  f16LowerLimit_Q : Ground
  f16UGain : Ground
  f16UpperLimit_D : Ground
  f16UpperLimit_Q : Ground
  f16WIGain : Ground
  f32Acc_D : Ground
  f32Acc_D_Out : Terminator
  f32Acc_Q : Ground
  f32Acc_Q_Out : Terminator
  f32IObsrvIn_1L_D : Ground
  f32IObsrvIn_1L_D_Out : Terminator
  f32IObsrvIn_1L_Q : Ground
  f32IObsrvIn_1L_Q_Out : Terminator
  f32IObsrv_D : Ground
  f32IObsrv_D_Out : Terminator
  f32IObsrv_Q : Ground
  f32IObsrv_Q_Out : Terminator
  s16Shift : Ground
  u16NShift : Ground
  f16PhaseErr : Outport
  wires:
  AMCLIB_BemfObsrvDQ_SF/13 -> f32IObsrv_Q_Out/1
  AMCLIB_BemfObsrvDQ_SF/12 -> f32IObsrv_D_Out/1
  AMCLIB_BemfObsrvDQ_SF/11 -> f16IObsrvIn_1H_Q_Out/1
  AMCLIB_BemfObsrvDQ_SF/10 -> f32IObsrvIn_1L_Q_Out/1
  AMCLIB_BemfObsrvDQ_SF/9 -> f16IObsrvIn_1H_D_Out/1
  AMCLIB_BemfObsrvDQ_SF/8 -> f32IObsrvIn_1L_D_Out/1
  AMCLIB_BemfObsrvDQ_SF/7 -> f16InErrK1_Q_Out/1
  AMCLIB_BemfObsrvDQ_SF/6 -> f32Acc_Q_Out/1
  AMCLIB_BemfObsrvDQ_SF/5 -> f16InErrK1_D_Out/1
  AMCLIB_BemfObsrvDQ_SF/4 -> f32Acc_D_Out/1
  AMCLIB_BemfObsrvDQ_SF/3 -> f16EObsrv_Q_Out/1
  AMCLIB_BemfObsrvDQ_SF/2 -> f16EObsrv_D_Out/1
  AMCLIB_BemfObsrvDQ_SF/1 -> f16PhaseErr/1
  f32IObsrv_Q/1 -> AMCLIB_BemfObsrvDQ_SF/28
  f32IObsrv_D/1 -> AMCLIB_BemfObsrvDQ_SF/27
  f16IObsrvIn_1H_Q/1 -> AMCLIB_BemfObsrvDQ_SF/26
  f32IObsrvIn_1L_Q/1 -> AMCLIB_BemfObsrvDQ_SF/25
  f16IObsrvIn_1H_D/1 -> AMCLIB_BemfObsrvDQ_SF/24
  f32IObsrvIn_1L_D/1 -> AMCLIB_BemfObsrvDQ_SF/23
  f16InErrK1_Q/1 -> AMCLIB_BemfObsrvDQ_SF/22
  f32Acc_Q/1 -> AMCLIB_BemfObsrvDQ_SF/21
  f16InErrK1_D/1 -> AMCLIB_BemfObsrvDQ_SF/20
  f32Acc_D/1 -> AMCLIB_BemfObsrvDQ_SF/19
  u16NShift/1 -> AMCLIB_BemfObsrvDQ_SF/18
  f16LowerLimit_Q/1 -> AMCLIB_BemfObsrvDQ_SF/17
  f16UpperLimit_Q/1 -> AMCLIB_BemfObsrvDQ_SF/16
  f16CC2sc_Q/1 -> AMCLIB_BemfObsrvDQ_SF/15
  f16CC1sc_Q/1 -> AMCLIB_BemfObsrvDQ_SF/14
  f16LowerLimit_D/1 -> AMCLIB_BemfObsrvDQ_SF/13
  f16UpperLimit_D/1 -> AMCLIB_BemfObsrvDQ_SF/12
  f16CC2sc_D/1 -> AMCLIB_BemfObsrvDQ_SF/11
  f16CC1sc_D/1 -> AMCLIB_BemfObsrvDQ_SF/10
  s16Shift/1 -> AMCLIB_BemfObsrvDQ_SF/9
  f16EGain/1 -> AMCLIB_BemfObsrvDQ_SF/8
  f16WIGain/1 -> AMCLIB_BemfObsrvDQ_SF/7
  f16UGain/1 -> AMCLIB_BemfObsrvDQ_SF/6
  f16IGain/1 -> AMCLIB_BemfObsrvDQ_SF/5
  f16Phase/1 -> AMCLIB_BemfObsrvDQ_SF/4
  f16Velocity/1 -> AMCLIB_BemfObsrvDQ_SF/3
  pUAB/1 -> AMCLIB_BemfObsrvDQ_SF/2
  pIAB/1 -> AMCLIB_BemfObsrvDQ_SF/1

== system ammclib_bam_S32K14x/AMCLIB/F16/AMCLIB_CurrentLoop_F16 ==
  f16UDcBus : Inport  OutDataTypeStr=int16
  pIDQReq : Inport  Port=2  OutDataTypeStr=Bus: SWLIBS_2Syst_F16  BusOutputAsStruct=on
  pIDQFbck : Inport  Port=3  OutDataTypeStr=Bus: SWLIBS_2Syst_F16  BusOutputAsStruct=on
  f16ControllerPIrAWDOut_preset : Inport  Port=4  OutDataTypeStr=int16
  f16ControllerPIrAWQOut_preset : Inport  Port=5  OutDataTypeStr=int16
  Reset : ResetPort  DisableCoverage=on
  AMCLIB_CurrentLoop_SF : S-Function  FunctionName=AMCLIB_CurrentLoop_SF_F16  Parameters=showStates,resetStatesEnable,f16CC1sc_D,f16CC2sc_D,u16NShift_D,f16CC1sc_Q,f16CC2sc_Q,u16NShift_Q  SFunctionDeploymentMode=off  EnableBusSupport=off
  copyright : Subsystem
      mask Display: text(10,90,'FILE:');text(10,75,'DESRIPTION:');text(10,60,'COPYRIGHT:');text(10,45,'VERSION:');text(10,30,'DATE:')
  copyright2 : Subsystem
      mask Display: text(10,90,'AMCLIB_CurrentLoop_BAM_F16.mdl');text(10,75,'PMSM Current Loop.');text(10,60,'NXP 2020');text(10,45,'1.0');text(10,30,'28-Mar-2020');
  f16CC1sc_D : Ground
  f16CC1sc_Q : Ground
  f16CC2sc_D : Ground
  f16CC2sc_Q : Ground
  f16InErrK1_D : Ground
  f16InErrK1_D_Out : Terminator
  f16InErrK1_Q : Ground
  f16InErrK1_Q_Out : Terminator
  f32Acc_D : Ground
  f32Acc_D_Out : Terminator
  f32Acc_Q : Ground
  f32Acc_Q_Out : Terminator
  u16NShift_D : Ground
  u16NShift_Q : Ground
  pUDQReq : Outport
  wires:
  AMCLIB_CurrentLoop_SF/5 -> f16InErrK1_Q_Out/1
  AMCLIB_CurrentLoop_SF/4 -> f32Acc_Q_Out/1
  AMCLIB_CurrentLoop_SF/3 -> f16InErrK1_D_Out/1
  AMCLIB_CurrentLoop_SF/2 -> f32Acc_D_Out/1
  AMCLIB_CurrentLoop_SF/1 -> pUDQReq/1
  f16InErrK1_Q/1 -> AMCLIB_CurrentLoop_SF/15
  f32Acc_Q/1 -> AMCLIB_CurrentLoop_SF/14
  f16InErrK1_D/1 -> AMCLIB_CurrentLoop_SF/13
  f32Acc_D/1 -> AMCLIB_CurrentLoop_SF/12
  u16NShift_Q/1 -> AMCLIB_CurrentLoop_SF/11
  f16CC2sc_Q/1 -> AMCLIB_CurrentLoop_SF/10
  f16CC1sc_Q/1 -> AMCLIB_CurrentLoop_SF/9
  u16NShift_D/1 -> AMCLIB_CurrentLoop_SF/8
  f16CC2sc_D/1 -> AMCLIB_CurrentLoop_SF/7
  f16CC1sc_D/1 -> AMCLIB_CurrentLoop_SF/6
  f16ControllerPIrAWQOut_preset/1 -> AMCLIB_CurrentLoop_SF/5
  f16ControllerPIrAWDOut_preset/1 -> AMCLIB_CurrentLoop_SF/4
  pIDQFbck/1 -> AMCLIB_CurrentLoop_SF/3
  pIDQReq/1 -> AMCLIB_CurrentLoop_SF/2
  f16UDcBus/1 -> AMCLIB_CurrentLoop_SF/1

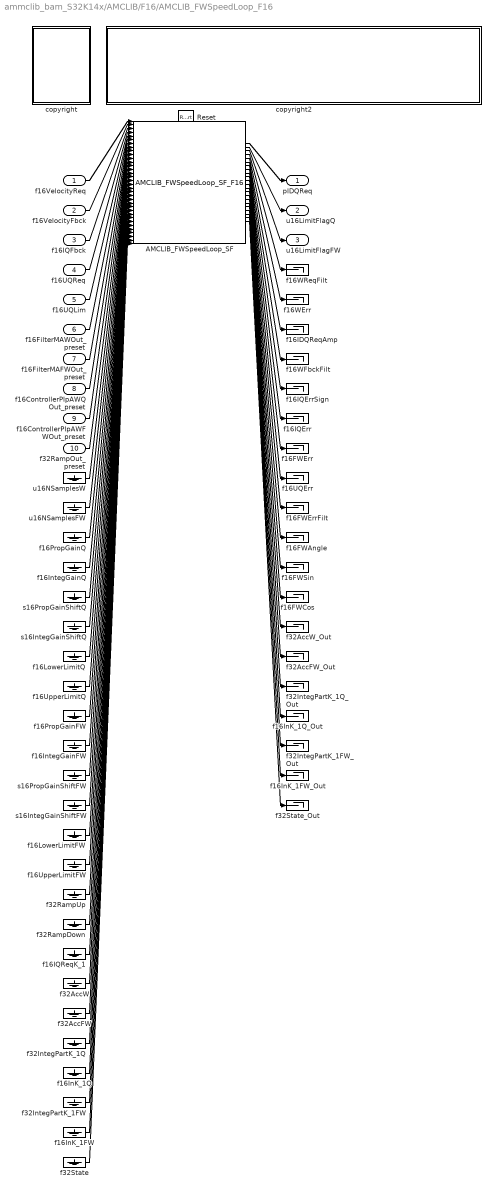
== system ammclib_bam_S32K14x/AMCLIB/F16/AMCLIB_FWSpeedLoop_F16 ==
  f16VelocityReq : Inport  OutDataTypeStr=int16
  f16VelocityFbck : Inport  Port=2  OutDataTypeStr=int16
  f16IQFbck : Inport  Port=3  OutDataTypeStr=int16
  f16UQReq : Inport  Port=4  OutDataTypeStr=int16
  f16UQLim : Inport  Port=5  OutDataTypeStr=int16
  f16FilterMAWOut_preset : Inport  Port=6  OutDataTypeStr=int16
  f16FilterMAFWOut_preset : Inport  Port=7  OutDataTypeStr=int16
  f16ControllerPIpAWQOut_preset : Inport  Port=8  OutDataTypeStr=int16
  f16ControllerPIpAWFWOut_preset : Inport  Port=9  OutDataTypeStr=int16
  f32RampOut_preset : Inport  Port=10  OutDataTypeStr=int32
  Reset : ResetPort  DisableCoverage=on
  AMCLIB_FWSpeedLoop_SF : S-Function  FunctionName=AMCLIB_FWSpeedLoop_SF_F16  Parameters=showStates,resetStatesEnable,showDebugOutputs,u16NSamplesW,u16NSamplesFW,f16PropGainQ,f16IntegGainQ,s16PropGainShiftQ,s16IntegGainShiftQ,f16LowerLimitQ,f16UpperLimitQ,f16PropGainFW,f16IntegGainFW,s16PropGainShiftFW,s16IntegGainShiftFW,f16LowerLimitFW,f16UpperLimitFW,f32RampUp,f32RampDown  SFunctionDeploymentMode=off  EnableBusSupport=off
  copyright : Subsystem
      mask Display: text(10,90,'FILE:');text(10,75,'DESRIPTION:');text(10,60,'COPYRIGHT:');text(10,45,'VERSION:');text(10,30,'DATE:')
  copyright2 : Subsystem
      mask Display: text(10,90,'AMCLIB_FWSpeedLoop_BAM_F16.mdl');text(10,75,'PMSM Speed Loop with Field Weakening.');text(10,60,'NXP 2020');text(10,45,'1.0');text(10,30,'28-Mar-2020');
  f16FWAngle : Terminator
  f16FWCos : Terminator
  f16FWErr : Terminator
  f16FWErrFilt : Terminator
  f16FWSin : Terminator
  f16IDQReqAmp : Terminator
  f16IQErr : Terminator
  f16IQErrSign : Terminator
  f16IQReqK_1 : Ground
  f16InK_1FW : Ground
  f16InK_1FW_Out : Terminator
  f16InK_1Q : Ground
  f16InK_1Q_Out : Terminator
  f16IntegGainFW : Ground
  f16IntegGainQ : Ground
  f16LowerLimitFW : Ground
  f16LowerLimitQ : Ground
  f16PropGainFW : Ground
  f16PropGainQ : Ground
  f16UQErr : Terminator
  f16UpperLimitFW : Ground
  f16UpperLimitQ : Ground
  f16WErr : Terminator
  f16WFbckFilt : Terminator
  f16WReqFilt : Terminator
  f32AccFW : Ground
  f32AccFW_Out : Terminator
  f32AccW : Ground
  f32AccW_Out : Terminator
  f32IntegPartK_1FW : Ground
  f32IntegPartK_1FW_Out : Terminator
  f32IntegPartK_1Q : Ground
  f32IntegPartK_1Q_Out : Terminator
  f32RampDown : Ground
  f32RampUp : Ground
  f32State : Ground
  f32State_Out : Terminator
  s16IntegGainShiftFW : Ground
  s16IntegGainShiftQ : Ground
  s16PropGainShiftFW : Ground
  s16PropGainShiftQ : Ground
  u16NSamplesFW : Ground
  u16NSamplesW : Ground
  pIDQReq : Outport
  u16LimitFlagQ : Outport  Port=2
  u16LimitFlagFW : Outport  Port=3
  wires:
  AMCLIB_FWSpeedLoop_SF/22 -> f32State_Out/1
  AMCLIB_FWSpeedLoop_SF/21 -> f16InK_1FW_Out/1
  AMCLIB_FWSpeedLoop_SF/20 -> f32IntegPartK_1FW_Out/1
  AMCLIB_FWSpeedLoop_SF/19 -> f16InK_1Q_Out/1
  AMCLIB_FWSpeedLoop_SF/18 -> f32IntegPartK_1Q_Out/1
  AMCLIB_FWSpeedLoop_SF/17 -> f32AccFW_Out/1
  AMCLIB_FWSpeedLoop_SF/16 -> f32AccW_Out/1
  AMCLIB_FWSpeedLoop_SF/15 -> f16FWCos/1
  AMCLIB_FWSpeedLoop_SF/14 -> f16FWSin/1
  AMCLIB_FWSpeedLoop_SF/13 -> f16FWAngle/1
  AMCLIB_FWSpeedLoop_SF/12 -> f16FWErrFilt/1
  AMCLIB_FWSpeedLoop_SF/11 -> f16UQErr/1
  AMCLIB_FWSpeedLoop_SF/10 -> f16FWErr/1
  AMCLIB_FWSpeedLoop_SF/9 -> f16IQErr/1
  AMCLIB_FWSpeedLoop_SF/8 -> f16IQErrSign/1
  AMCLIB_FWSpeedLoop_SF/7 -> f16WFbckFilt/1
  AMCLIB_FWSpeedLoop_SF/6 -> f16IDQReqAmp/1
  AMCLIB_FWSpeedLoop_SF/5 -> f16WErr/1
  AMCLIB_FWSpeedLoop_SF/4 -> f16WReqFilt/1
  AMCLIB_FWSpeedLoop_SF/3 -> u16LimitFlagFW/1
  AMCLIB_FWSpeedLoop_SF/2 -> u16LimitFlagQ/1
  AMCLIB_FWSpeedLoop_SF/1 -> pIDQReq/1
  f32State/1 -> AMCLIB_FWSpeedLoop_SF/34
  f16InK_1FW/1 -> AMCLIB_FWSpeedLoop_SF/33
  f32IntegPartK_1FW/1 -> AMCLIB_FWSpeedLoop_SF/32
  f16InK_1Q/1 -> AMCLIB_FWSpeedLoop_SF/31
  f32IntegPartK_1Q/1 -> AMCLIB_FWSpeedLoop_SF/30
  f32AccFW/1 -> AMCLIB_FWSpeedLoop_SF/29
  f32AccW/1 -> AMCLIB_FWSpeedLoop_SF/28
  f16IQReqK_1/1 -> AMCLIB_FWSpeedLoop_SF/27
  f32RampDown/1 -> AMCLIB_FWSpeedLoop_SF/26
  f32RampUp/1 -> AMCLIB_FWSpeedLoop_SF/25
  f16UpperLimitFW/1 -> AMCLIB_FWSpeedLoop_SF/24
  f16LowerLimitFW/1 -> AMCLIB_FWSpeedLoop_SF/23
  s16IntegGainShiftFW/1 -> AMCLIB_FWSpeedLoop_SF/22
  s16PropGainShiftFW/1 -> AMCLIB_FWSpeedLoop_SF/21
  f16IntegGainFW/1 -> AMCLIB_FWSpeedLoop_SF/20
  f16PropGainFW/1 -> AMCLIB_FWSpeedLoop_SF/19
  f16UpperLimitQ/1 -> AMCLIB_FWSpeedLoop_SF/18
  f16LowerLimitQ/1 -> AMCLIB_FWSpeedLoop_SF/17
  s16IntegGainShiftQ/1 -> AMCLIB_FWSpeedLoop_SF/16
  s16PropGainShiftQ/1 -> AMCLIB_FWSpeedLoop_SF/15
  f16IntegGainQ/1 -> AMCLIB_FWSpeedLoop_SF/14
  f16PropGainQ/1 -> AMCLIB_FWSpeedLoop_SF/13
  u16NSamplesFW/1 -> AMCLIB_FWSpeedLoop_SF/12
  u16NSamplesW/1 -> AMCLIB_FWSpeedLoop_SF/11
  f32RampOut_preset/1 -> AMCLIB_FWSpeedLoop_SF/10
  f16ControllerPIpAWFWOut_preset/1 -> AMCLIB_FWSpeedLoop_SF/9
  f16ControllerPIpAWQOut_preset/1 -> AMCLIB_FWSpeedLoop_SF/8
  f16FilterMAFWOut_preset/1 -> AMCLIB_FWSpeedLoop_SF/7
  f16FilterMAWOut_preset/1 -> AMCLIB_FWSpeedLoop_SF/6
  f16UQLim/1 -> AMCLIB_FWSpeedLoop_SF/5
  f16UQReq/1 -> AMCLIB_FWSpeedLoop_SF/4
  f16IQFbck/1 -> AMCLIB_FWSpeedLoop_SF/3
  f16VelocityFbck/1 -> AMCLIB_FWSpeedLoop_SF/2
  f16VelocityReq/1 -> AMCLIB_FWSpeedLoop_SF/1
